simulink model "simullink_model_COLMS"  (R2022a)
settings: Solver=VariableStepAuto  StartTime=0.0  StopTime=250.0  RelTol=1e-3
settings Model: Creator=MattiP  LastModifiedBy=loreb
settings DebuggingCC: UnconnectedInputMsg=warning  UnconnectedOutputMsg=warning  UnconnectedLineMsg=warning
settings RTWCC: DLArmComputeVersion=19.05

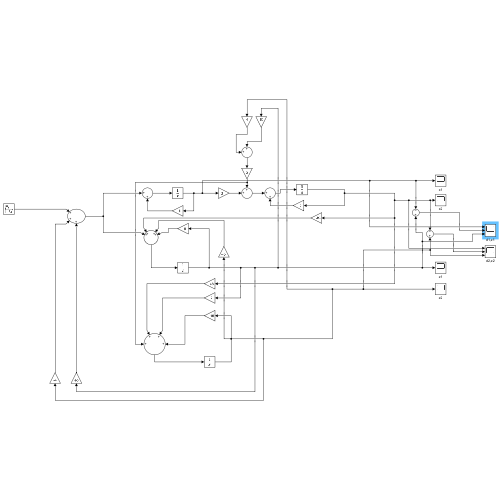
[thumbnail: Simulink's stored preview of the top-level diagram]
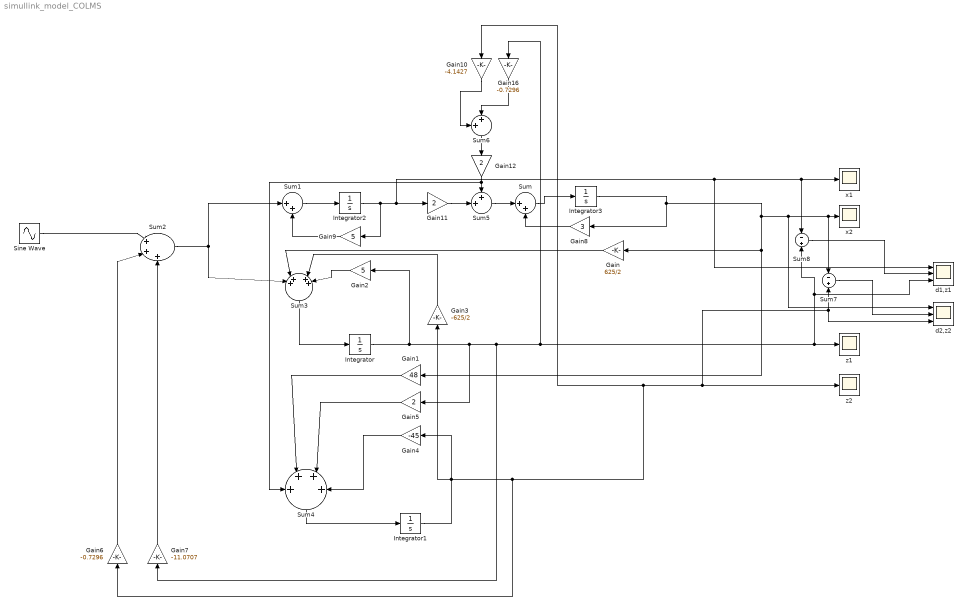
== system simullink_model_COLMS ==
  Gain : Gain  Gain=625/2
  Gain1 : Gain  Gain=48
  Gain10 : Gain  Gain=-4.1427
  Gain11 : Gain  Gain=2
  Gain12 : Gain  Gain=2
  Gain16 : Gain  Gain=-0.7296
  Gain2 : Gain  Gain=5
  Gain3 : Gain  Gain=-625/2
  Gain4 : Gain  Gain=-45
  Gain5 : Gain  Gain=2
  Gain6 : Gain  Gain=-0.7296
  Gain7 : Gain  Gain=-11.0707
  Gain8 : Gain  Gain=3
  Gain9 : Gain  Gain=5
  Integrator : Integrator  InitialCondition=10
  Integrator1 : Integrator  InitialCondition=19
  Integrator2 : Integrator  InitialCondition=-30  ZeroCross=off
  Integrator3 : Integrator  InitialCondition=25  ZeroCross=off
  Sine Wave : Sin  Amplitude=10  Frequency=0.1  SampleTime=0
  Sum : Sum  Inputs=|++
  Sum1 : Sum  Inputs=|++
  Sum2 : Sum  Inputs=|+++
  Sum3 : Sum  Inputs=|++||++|
  Sum4 : Sum  Inputs=+|+|+|+
  Sum5 : Sum  Inputs=++|
  Sum6 : Sum  Inputs=++|
  Sum7 : Sum  Inputs=-+
  Sum8 : Sum  Inputs=-+
  d1,z1 : Scope  NumInputPorts=3
  d2,z2 : Scope  NumInputPorts=3
  x1 : Scope
  x2 : Scope
  z1 : Scope
  z2 : Scope
  wires:
  Gain/1 -> Sum3/2
  Sum3/1 -> Integrator/1
  Sum4/1 -> Integrator1/1
  Gain1/1 -> Sum4/2
  Gain3/1 -> Sum3/3
  Gain5/1 -> Sum4/3
  Gain8/1 -> Sum/2
  Gain7/1 -> Sum2/3
  Gain6/1 -> Sum2/2
  Sum2/1 -> Sum1/1, Sum3/1
  Sum1/1 -> Integrator2/1
  Sum/1 -> Integrator3/1
  Gain11/1 -> Sum5/2
  Integrator1/1 -> Gain10/1, Sum7/2, d2,z2/3, z2/1, Gain6/1, Gain3/1, Gain4/1
  Gain10/1 -> Sum6/1
  Gain16/1 -> Sum6/2
  Sum6/1 -> Gain12/1
  Gain12/1 -> Sum4/1, Sum5/1
  Sine Wave/1 -> Sum2/1
  Gain4/1 -> Sum4/4
  Gain9/1 -> Sum1/2
  Gain2/1 -> Sum3/4
  Sum5/1 -> Sum/1
  Sum8/1 -> d1,z1/2
  Integrator/1 -> Gain2/1, Sum8/2, d1,z1/3, z1/1, Gain16/1, Gain7/1, Gain5/1
  Integrator2/1 -> Gain9/1, d1,z1/1, Sum8/1, x1/1, Gain11/1
  Sum7/1 -> d2,z2/2
  Integrator3/1 -> d2,z2/1, Sum7/1, x2/1, Gain1/1, Gain/1, Gain8/1
